simulink model "DoD_simulink_model"  (R2018a)
settings: Solver=VariableStepAuto  StartTime=0.0  StopTime=tsim  RelTol=1e-3
values from neighbouring files (symbols this model uses):
  Aineq = [eye(N_MPC);-eye(N_MPC)]    [Copy_of_DoD_simulation.m]    (also in DoD_simulation.m)
  bineq = [fracU_max; -fracU_min]    [Copy_of_DoD_simulation.m]    (also in DoD_simulation.m)
  Gamma = WW.'*[(BB.'*QQ + SS.')*(AA + BB*EE) + (BB.'*SS + RR)*EE, -(BB.'*QQ + SS.')*kron(ones(N_MPC+1,1),NN)]    [Copy_of_DoD_simulation.m]    (also in DoD_simulation.m)
  Linv = L_H\eye(size(H,1))    [Copy_of_DoD_simulation.m]    (also in DoD_simulation.m)
  n_in = size(Bcd,2)    [Copy_of_DoD_simulation.m]    (also in DoD_simulation.m)
  n_out = size(Cc,1)    [Copy_of_DoD_simulation.m]    (also in DoD_simulation.m)
  opt = mpcqpsolverOptions    [Copy_of_DoD_simulation.m]    (also in DoD_simulation.m)
  phi0 = 10*(pi/180)    (= 0.174532925199)    [Copy_of_DoD_simulation.m]    (also in DoD_simulation.m = 0.0349065850399)
  T = 0.01    [Copy_of_DoD_simulation.m]    (also in DoD_simulation.m)
  theta0 = 10*(pi/180)    (= 0.174532925199)    [Copy_of_DoD_simulation.m]    (also in DoD_simulation.m = 0)
undefined symbols (not defined in the file or in its folder): Acd, Bcd
settings Model: Creator=timot  LastModifiedBy=timot

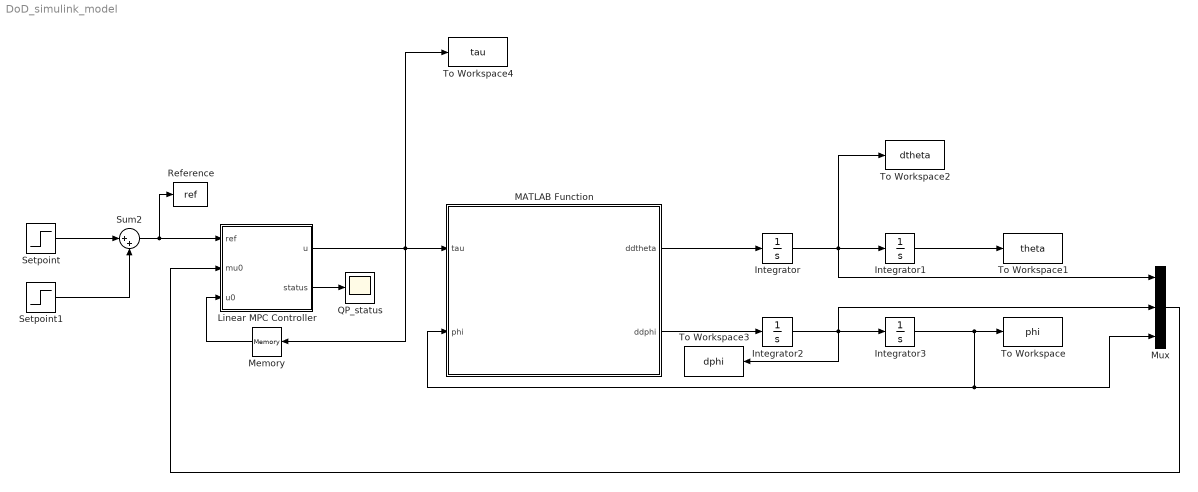
== system DoD_simulink_model ==
  Integrator : Integrator
  Integrator1 : Integrator  InitialCondition=theta0
  Integrator2 : Integrator
  Integrator3 : Integrator  InitialCondition=phi0
  Linear MPC Controller : MATLAB Function  TreatAsAtomicUnit=on  SystemSampleTime=T
  MATLAB Function : MATLAB Function  TreatAsAtomicUnit=on
  Memory : Memory  InitialCondition=zeros(n_out,1)  InheritSampleTime=on
  Mux : Mux  Inputs=3
  QP_status : Scope
  Reference : ToWorkspace  VariableName=ref  SaveFormat=Structure With Time  SampleTime=-1
  Setpoint : Step  Time=10  SampleTime=0
  Setpoint1 : Step  Time=20  After=-1  SampleTime=0
  Sum2 : Sum  Inputs=|++
  To Workspace : ToWorkspace  VariableName=phi  SaveFormat=Structure With Time  SampleTime=-1
  To Workspace1 : ToWorkspace  VariableName=theta  SaveFormat=Structure With Time  SampleTime=-1
  To Workspace2 : ToWorkspace  VariableName=dtheta  SaveFormat=Structure With Time  SampleTime=-1
  To Workspace3 : ToWorkspace  VariableName=dphi  SaveFormat=Structure With Time  SampleTime=-1
  To Workspace4 : ToWorkspace  VariableName=tau  SaveFormat=Structure With Time  SampleTime=-1
  wires:
  MATLAB Function/1(ddtheta) -> Integrator/1
  Integrator/1 -> Integrator1/1, Mux/1, To Workspace2/1
  MATLAB Function/2(ddphi) -> Integrator2/1
  Integrator2/1 -> Mux/2, To Workspace3/1, Integrator3/1
  Integrator1/1 -> To Workspace1/1
  Integrator3/1 -> Mux/3, MATLAB Function/2(phi), To Workspace/1
  Linear MPC Controller/1(u) -> MATLAB Function/1(tau), Memory/1, To Workspace4/1
  Memory/1 -> Linear MPC Controller/3(u0)
  Linear MPC Controller/2(status) -> QP_status/1
  Sum2/1 -> Reference/1, Linear MPC Controller/1(ref)
  Mux/1 -> Linear MPC Controller/2(mu0)
  Setpoint1/1 -> Sum2/2
  Setpoint/1 -> Sum2/1

== matlab function DoD_simulink_model/Linear MPC Controller ==
  settings: updateMethod=DISCRETE  sampleTime=T
  data: ref input; u output size=1; mu0 input; Linv parameter; opt parameter; n_in parameter size=1; u0 input; status output; Gamma parameter; Acd parameter; Bcd parameter; Aineq parameter; bineq parameter
function [u, status] = MPC(ref, mu0, Linv, opt, n_in, u0, Gamma, Acd, Bcd, Aineq, bineq)
%#codegen

% Predict state at next time step
mu1 = Acd*mu0 + Bcd*u0;

% Compute linear coefficient of QP
kk = [mu1; u0; ref];
g = Gamma*kk;

iA0 = false(size(Aineq,1),1);   % Initial active constraints

% The KWIK algorithm defines inequality constraints as Ax >= b rather than 
% Ax <= b, as in the quadprog command.
[uMPC, status] = mpcqpsolver(Linv, g, -Aineq, -bineq, [], zeros(0,1), iA0, opt);

% Return next control action
u = uMPC(1:n_in);

== matlab function DoD_simulink_model/MATLAB Function ==
  data: tau input; ddtheta output; ddphi output; MM parameter; phi input
function [ddtheta, ddphi] = DoDPlantModel(tau,MM, phi)



%Parameters
mo = 1.5;           % kg
mh = 1.0;           % kg

ro = 0.1;           % m
rh = 0.2;           % m

g = 9.8;            % m/s^2




gq = [0; -mo*g*(rh + ro)*sin(phi)];


out = MM\(tau - gq);
ddtheta = out(1);
ddphi = out(2);
